simulink model "SimulationModel"  (R2017b)
settings: Solver=ode4  StartTime=0.0  StopTime=inf  RelTol=1e-3
PreLoadFcn:
  | addLibrariesInPath('sim')
PostLoadFcn:
  | loadRobotParameters
StartFcn:
  | simApp = SimDisplay.getInstance;
  | simApp.reset;
  | simApp.TrackView.setup(double(SitesPositions), ObstaclesPositions,ObstaclesVertices,ObstaclesEdges);
values from neighbouring files (symbols this model uses):
  AngularSpeed = 300    [loadRobotParameters.m]
  AxleLength = 16.7    [loadRobotParameters.m]
  DISTANCE_APPROACH = 45    [loadRobotParameters.m]
  DISTANCE_MAX = 200    [loadRobotParameters.m]
  DISTANCE_PARKING = 10    [loadRobotParameters.m]
  do_one_run = true    [loadRobotParameters.m]
  EncL_init = 0    [loadRobotParameters.m]
  EncR_init = 0    [loadRobotParameters.m]
  EncRes = 636    [loadRobotParameters.m]
  lcam = [21, 90]    [loadRobotParameters.m]
  motorL = [-967.207000 -900.359000 -783.375000 -618.344000 -325.884000 -0.000000 0.000000 325.884000 618.344000 783.375000 900.359000 967.207000 ]    [loadRobotParameters.m]
  motorR = [-937.961000 -850.223000 -768.752000 -618.344000 -302.905000 -0.000000 0.000000 302.905000 618.344000 768.752000 850.223000 937.961000 ]    [loadRobotParameters.m]
  motorX = [-100.000000 -90.000000 -70.000000 -50.000000 -30.000000 -27.000000 27.000000 30.000000 50.000000 70.000000 90.000000 100.000000 ]    [loadRobotParameters.m]
  pcam = [24, 100]    [loadRobotParameters.m]
  RADIUS_TARGET = 5    [loadRobotParameters.m]
  S_ROT = 10    [loadRobotParameters.m]
  SPEED_APPROACH = 15    [loadRobotParameters.m]
  SPEED_BACK = 5    [loadRobotParameters.m]
  SPEED_NORMAL = 30    [loadRobotParameters.m]
  startPos = single([150 150])    [loadRobotParameters.m]
  TauMotor = 0.1    [loadRobotParameters.m]
  TH1 = 5    [loadRobotParameters.m]
  TH2 = 15    [loadRobotParameters.m]
  theta0 = 0    [loadRobotParameters.m]
  Ts = 0.1    [loadRobotParameters.m]
  WAIT_TIME = 4    [loadRobotParameters.m]
  WheelRadius = 7/2    (= 3.5)    [loadRobotParameters.m]
undefined symbols (not defined in the file or in its folder): ObstaclesEdges, ObstaclesVertices, SitesPositions
libraries: simulink_extras x2, simulink x2, Fuzzy_Type2_Lib x1, realtime_pacer_lib x1, cstblocks x1
(part 2 of 2)

== stateflow chart SimulationModel/RobotModel/Controller/FeedbackController/ControllerModesDistance ==
  state CurrentMove [parallel]
    settings: executionOrder=1
    state Normal
      entry:
      EncodersZero = Encoders;
      entry,during:
      CurrentDistance = CurrentMoveFcn(Encoders,EncodersZero);
    state distance = CurrentMoveFcn(enc,zero) [function]
    (default) -> Normal
    Normal -> Normal : Reset
  state ModeControl [parallel]
    settings: executionOrder=2
    state SpeedControl
      entry:
      CurrentMove.Reset;
      ResetDistancePI;
      DistanceError = Cmd.Position;
      PrevDistance = CurrentDistance;
      during:
      DistanceError = (Cmd.Position - (CurrentDistance-PrevDistance)/Ts);
      PrevDistance = CurrentDistance;
    state DistanceControl
      entry:
      CurrentMove.Reset;
      ResetDistancePI;
      entry,during:
      DistanceError = Cmd.Position - CurrentDistance;
    (default) -> (junction 73)
    (junction 73) -> (junction 72) [order 1] : [Cmd.Mode == EMode.SPEED]
    (junction 73) -> DistanceControl [order 2]
    (junction 72) -> SpeedControl
    SpeedControl -> DistanceControl : [Cmd.Mode == EMode.DISTANCE]
    DistanceControl -> SpeedControl : [Cmd.Mode == EMode.SPEED]
  state ResetIntegrator [parallel]
    settings: executionOrder=4
    (default) -> (junction 189) : {
        | PrevCmd = Cmd.Position;
        | PrevMode = Cmd.Mode;
        | }
    ResetIntegrator -> (junction 189)
    (junction 189) -> (junction 192) [order 1] : [Cmd.Mode ~= PrevMode]
    (junction 189) -> (junction 179) [order 2]
    (junction 192) -> (junction 185)
    (junction 179) -> (junction 185) [order 1] : [sign(Cmd.Position) ~= sign(PrevCmd)]
    (junction 179) -> (junction 188) [order 2]
    (junction 185) -> (junction 187) : {
        | ResetDistancePI;
        | }
    (junction 187) -> (junction 188)
    (junction 188) -> (junction 181) : {
        | PrevCmd = Cmd.Position;
        | PrevMode = Cmd.Mode;
        | }
  state ErrorInitialCondition [parallel]
    settings: executionOrder=3
    (default) -> (junction 170)
    ErrorInitialCondition -> (junction 170)
    (junction 170) -> (junction 171) [order 1] : [abs(DistanceError) < 30 && ...
        | abs(Cmd.Angle) < 1 && ...
        | Cmd.Mode == EMode.SPEED]
    (junction 170) -> (junction 172) [order 2] : {
        | DistanceIC = single(0);
        | }
    (junction 171) -> (junction 173) : {
        | DistanceIC = 30 * sign(Cmd.Position) - DistanceError;
        | }
    (junction 173) -> (junction 172)
    (junction 172) -> (junction 174)
  data: enc function_input int32 size=2; zero function_input int32 size=2; distance function_output; EncodersZero local int32 size=2; PrevDistance local; PrevCmd local; PrevMode local; Encoders input int32 size=2; CurrentDistance local single; DistanceError output single size=1; Cmd input Bus: bus_Command; Ts parameter; DistanceIC output
  events: Reset local FUNCTION_CALL_EVENT; ResetDistancePI output EITHER_EDGE_EVENT

== stateflow chart SimulationModel/Scoring/Referee/Referee ==
  state Standby
    entry:
    numTargets = size(SitesPositions,1);
    targetsFound = false(size(SitesPositions,1),1);
    timeLastTargetFound = 0;
    elapsedTime = 0;
    numTargetsFound = 0;
    allowedRunTime = 180;
    startingRadius = 10;
    targetBoundaryRadius = 7;
    statTimeReq = 2.5;
  state Running
    entry: startTiming;
    during:
    elapsedTime = getTiming;
    [nearLocation, currentTarget] = testIfNearLocation(robotPosition, SitesPositions, targetBoundaryRadius);
    state NearLocation
      entry: snapshotTime = elapsedTime;
    state Roaming
    Roaming -> NearLocation : [nearLocation == true]
    (default) -> Roaming
    NearLocation -> Roaming [order 2] : [nearLocation == false]
    NearLocation -> (junction 43) [order 1] : [(elapsedTime - snapshotTime) > statTimeReq]
    (junction 44) -> Roaming
    (junction 43) -> (junction 44) : {[targetsFound, timeLastTargetFound] = ...
        | updateTargetsFound(targetsFound, currentTarget, timeLastTargetFound,elapsedTime);
        | numTargetsFound = sum(targetsFound);}
  state Finished
  (default) -> Standby
  Finished -> Standby : [StartFlag == false]
  Standby -> Running : [StartFlag == true &&...
      | distancefrom(robotPosition, startPos) < startingRadius ]
  Running -> Standby [order 2] : [StartFlag == false]
  Running -> Finished [order 1] : [numTargetsFound == numTargets ||...
      |  elapsedTime >= allowedRunTime-sqrt(eps)]
  data: et function_output; tfound_in function_input; currentT function_input; tfound_out function_output; lastTime_in function_input; lastTime_out function_output; time function_input; robotPos function_input; targetPos function_input; proximityVal function_input; nearLoc function_output; currentLoc function_output; pos function_input; x0 function_input; d function_output; startPos parameter; allowedRunTime local; statTimeReq local; startingRadius local; robotPosition input; targetBoundaryRadius local; StartFlag input; SitesPositions parameter; timeLastTargetFound output; nearLocation local; numTargetsFound local; elapsedTime output; numTargets local; currentTarget local; targetsFound output; snapshotTime local; local_t local =0; sim_time input
  function startTiming:
    | function startTiming
    | global local_t sim_time
    | 
    | if strcmp(coder.target,'rtw')
    |     coder.ceval('tic',int32(2));
    | else
    |     local_t = sim_time;
    | end
  function et = getTiming:
    | function et = getTiming
    | global sim_time local_t
    | 
    | lt = 0;
    | 
    | if strcmp(coder.target,'rtw')
    |     coder.ceval('toc',coder.wref(lt),int32(2));
    | else
    |     lt = sim_time - local_t;
    | end
    | 
    | et = lt;
  function [tfound_out, lastTime_out] = updateTargetsFound(tfound_in, currentT, lastTime_in, time):
    | function [tfound_out, lastTime_out] = updateTargetsFound(tfound_in, currentT, lastTime_in, time)
    | 
    | if any(tfound_in & currentT) %is this an existing target
    |     lastTime_out = lastTime_in;
    | else
    |     lastTime_out = time;
    | end
    | 
    | tfound_out = tfound_in | currentT; %update list of found targets
  function [nearLoc, currentLoc] = testIfNearLocation(robotPos, targetPos, proximityVal):
    | function [nearLoc, currentLoc] = testIfNearLocation(robotPos, targetPos, proximityVal)
    | %#codegen
    | delta = bsxfun(@minus, targetPos, robotPos);
    | dist = sum(delta.^2,2);
    | 
    | currentLoc = dist <= proximityVal^2;
    | nearLoc = any(currentLoc);
  function d = distancefrom(pos,x0):
    | function d = distancefrom(pos,x0)
    | d = sqrt(sum((pos-x0).^2));

== matlab function SimulationModel/Scoring/FigureOutput/call_plotFigure ==
  data: X input; SitesPositions parameter; T_found input; t_last input; t input; T_located input; pcam parameter; lcam parameter; robotheta input; ArmAngleEstimated input; ArmAngleCommand input; DisplayPositions input
function fcn(X, SitesPositions, T_found, t_last, t, T_located,pcam,lcam,robotheta,...
    ArmAngleEstimated, ArmAngleCommand, DisplayPositions)
coder.extrinsic('plotFigure');

plotFigure(X, SitesPositions, T_found, t_last, t, T_located,pcam,lcam,robotheta,...
    single(ArmAngleEstimated), single(ArmAngleCommand), DisplayPositions);

== matlab function SimulationModel/RobotModel/Robot/Sensors Camera_Distance/Camera/relative_to_targets ==
  data: robotPos input size=[1 2]; robotTheta input size=1; dist output; bear output; SitesPositions parameter single; ObstaclesVertices parameter; ObstaclesEdges parameter; pcam parameter; lcam parameter
 function [dist,bear] = targets(robotPos,robotTheta,SitesPositions,ObstaclesVertices, ObstaclesEdges, pcam,lcam)
%#codegen
%% TARGETS Returns distance and bearing for each target relative tos robot
%
% Distances and positions are in cm
% Angles are in degrees
%
% Inputs
%   - hCam: Cam height (from ground)
%   - targetsPos: Position of targets (X,Y)
%   - robotPos: Robot position (X,Y)
%   - robotTheta: Robot angle
%
% Outputs
%   - dist (array nx1 with n=nb targets): Distances for each target,
%       if a target cannot be seen by the camera associated distance
%       is equal to -1
%   - bearing (array nx1 with n=nb targets): Angles for each target,
%       if a target cannot be seen by the camera associated angle is
%       equal to -1
%

% Get camera field of vision
% [pcam,lcam]=camera(hCam);
% betaCam = 21 ;
% etaCam = 27 ;
% [pcam, lcam] = cameraAnalytic(hCam,90-alphaCam, betaCam, etaCam);

% Convert target position to robot reference
[x,y] = world2robot(robotPos(1),robotPos(2),robotTheta,SitesPositions(:,1),SitesPositions(:,2));

% Convert Obstacles positions to robot reference
[vx,vy] = world2robot(robotPos(1),robotPos(2),robotTheta,ObstaclesVertices(:,1),ObstaclesVertices(:,2));

% Get left and right detector indicators
%[leftFlag, rightFlag] = isThereSomething(vx, vy, obstaclesEdges);

% Get distance and bearing for each point relative to robot
[distance,bearing] = isincamera(pcam,lcam,x,y,vx,vy,ObstaclesEdges);

% sort by descending order and return 6 elements
[distance,idxsort] = sort(distance,'descend');
bearing = bearing(idxsort);
if length(distance)<6
    dist = [distance;zeros(6-length(distance),1)];
    bear = [bearing;zeros(6-length(bearing),1)] ;
else
    dist = distance(1:6);
    bear = bearing(1:6);
end

end

function [x_new,y_new]=world2robot(x_robot,y_robot,theta_robot,x_world,y_world)
% WORLD2ROBOT Convert coordinates from world to robot
%
% Inputs
%   - x_robot: Robot X position (in world reference)
%   - y_robot: Robot Y position (in world reference)
%   - theta_robot: Robot angle  (in world reference)
%   - x_world: X value(s) to convert (in world reference)
%   - y_world: Y value(s) to convert (in world reference)
%
% Outpus
%   - x_new: Point(s) coordinate (X) in robot reference
%   - y_new: Point(s) coordinate (Y) in robot reference

% Translate coordinates reference
x_dif=x_world-x_robot;
y_dif=y_world-y_robot;

% Rotate coordinates reference
% x_new=x_dif*cosd(theta_robot)-y_dif*sind(theta_robot);
% y_new=x_dif*sind(theta_robot)+y_dif*cosd(theta_robot);
x_new = cosd(theta_robot)*x_dif + sind(theta_robot)*y_dif;
y_new = cosd(theta_robot)*y_dif - sind(theta_robot)*x_dif;
% see http://www.mathematics-online.org/inhalt/aussage/aussage444/

% TODO We have identified that the sign of converted coordinates is the
% opposite of the expected but we don't have an explanation for that
% x_new = -x_new;
% y_new = -y_new;

end

function [dist,bearing]=isincamera(p,l,x,y,vx,vy,OE)
%% ISINCAMERA Distance and angle from current robot position
%
% Inputs
%   - p (2 elements vector): Minimal and maximal depth for camera (Y axis)
%   - l (2 elements vector): Minimal and maximal width for camera (X axis)
%   - x (vector): X coordinate of point(s)
%   - y (vector): Y coordinate of point(s)
%
% Outputs
%   - dist (vector): Distance of each point from camera (robot), -1 if
%       point cannot be seen by camera.
%   - bearing (vector): Angle of each point from camera (robot), -1 if
%       point cannot be seen by camera.
%

% Calculate coefficients for lines that defines the camera field of vision
% Field vision limits in Y axis are constants (y = p(1) or y = p(2))
% c1=polyfit(p(1:2),[-l(1)/2 -l(2)/2],1);
% c2=polyfit(p(1:2),[l(1)/2 l(2)/2],1);

% To be visible a point must match all the following criterion
%   - Y >= minimal depth
%   - Y <= maximal depth
%   - X >= - (width for current Y) / 2
%   - X <=   (width for current Y) / 2
%

%isvisible = y>=p(1) & y<=p(2) & (x>=polyval(c1,y) & x<=polyval(c2,y));
% isvisible = x>=p(1) & x<=p(2) & (y>=polyval(c1,x) & y<=polyval(c2,x));

%TTx = [p(1) p(2) p(2) p(1)]' ;
%TTy = [l(1)/2 l(2)/2 -l(2)/2 -l(1)/2]' ;
%TTx = [[p(1); p(2); p(1)] [p(1); p(2); p(2)]];
%TTy = [[l(1)/2; l(2)/2; -l(1)/2] [-l(1)/2; l(2)/2; -l(2)/2]];
TTx = [p(1); p(2); p(2); p(1)];
TTy = [l(1)/2; l(2)/2; -l(2)/2; -l(1)/2];

[vpX, vpY] = CastRays(0, 0, [vx vy], OE);
vpX = vpX(2:end,:);
vpX = vpX(:);
vpY = vpY(2:end,:);
vpY = vpY(:);

%dis = simDisplay.getInstance;
%patch(vpX, vpY, zeros(size(vpX)), 'Parent', dis.TrackView.Axes);


isvisible = true(size(x));
for k=1:length(isvisible)
    isvisible(k) = any(myInpolygon(x(k), y(k), TTx, TTy)) && ...
        any(myInpolygon(x(k), y(k), vpX, vpY));
%     isvisible(k) = any(inTriangle(x(k), y(k), TTx, TTy)) &&...
%         any(inTriangle(x(k), y(k), vpX, vpY));
end

% Calculate distance and bearing for all points
dist = sqrt(x.^2 + y.^2);
% bearing = atan2d(y,x);
bearing = atan2d(x,-y)-90;

% Replace values by -1 for points that are not visible
dist(~isvisible) = 0;
bearing(~isvisible) = 0;

end

function [vpX, vpY] = CastRays(x, y, vertices, edges)
% Cast rays

vertices = [vertices zeros(length(vertices),5)];
% Compute relative cartesian coordinates
vertices(:,3) = vertices(:,1) -...
    x;

vertices(:,4) = vertices(:,2) -...
    y;


% Compute relative polar coordinates
[vertices(:,5), vertices(:,6)] =...
    cart2pol(vertices(:,3), vertices(:,4));

vertices(:,5) = mod(vertices(:,5), 2*pi);


% Sort rows by angle and get reverse permutation
[vertices, ind] = sortrows(vertices, 5);

[~, ind] = sort(ind, 'ascend');


% Modify the edges indices accordingly
edges(:,1) = ind(edges(:,1));

edges(:,2) = ind(edges(:,2));


% Ensure that the left vertex of each edge is on the left
Tdiff = vertices(edges(:,1),5) -...
    vertices(edges(:,2),5);

ind = xor(Tdiff < 0, abs(Tdiff)>pi);

edges(ind, [1 2]) =...
    edges(ind, [2 1]);

vpX = zeros(3, size(vertices,1));
vpY = zeros(3, size(vertices,1));


% Loop over each vertex and get the left vertex of the
% right triangle and the right edge of the left triangle
for ray = 1:size(vertices,1)
    
    % Find edges that cross the ray
    TdiffL = vertices(edges(:,1),5) -...
        vertices(ray,5);
    TdiffR = vertices(ray,5) -...
        vertices(edges(:,2),5);
    intersects = find(xor(TdiffL >= 0, abs(TdiffL)>pi) &...
        xor(TdiffR >= 0, abs(TdiffR)>pi));
    
    
    % Compute intersection coordinates
    [~, ~, interX, interY] = lineSegmentsIntersection(x, y, vertices(ray,1),...
        vertices(ray,2), vertices(edges(intersects,1),1),...
        vertices(edges(intersects,1),2), vertices(edges(intersects,2),1),...
        vertices(edges(intersects,2),2));
    
    
    % Sort the intersections (coordinates and index of the
    % edges) by distance to viewpoint
    [~, dist2vp] = cart2pol(interX - x, interY - y);
    
    [~,ind] = sort(dist2vp, 'ascend');
    
    intersects = intersects(ind);
    
    
    % Pick the first intersection, with the exception that it
    % must not be a right edge for the left triangle or a left
    % edge for the right triangle. Assign the result
    leftInd = find(edges(intersects,2) ~= ray, 1, 'first');
    rightInd = find(edges(intersects,1) ~= ray, 1, 'first');
    if isempty(leftInd)
        leftInd = 1;
    end
    if isempty(rightInd)
        rightInd = 1;
    end
    rightInd = rightInd(1);
    leftInd = leftInd(1);
    
    vpX(1,ray) = x;
    vpY(1,ray) = y;
    
    vpX(2,ray) = interX(ind(rightInd));
    vpY(2,ray) = interY(ind(rightInd));
    
    indBack = mod(ray-2, size(vertices,1))+1;
    vpX(3,indBack) = interX(ind(leftInd));
    vpY(3,indBack) = interY(ind(leftInd));
    
end

end

== matlab function SimulationModel/RobotModel/Robot/Sensors Camera_Distance/Camera/dist_bearing2locatedTargets ==
  data: robotPos input; dist input; locatedTargets output; bearing input; robotTheta input
function locatedTargets = fcn(robotPos, dist, bearing, robotTheta)
%#codegen

loc = dist > 0;

locatedTargetsX = zeros(size(dist));
locatedTargetsY = locatedTargetsX;

targetTheta = robotTheta + bearing(loc);

locatedTargetsX(loc) = robotPos(1) + dist(loc) .* cosd(targetTheta);
locatedTargetsY(loc) = robotPos(2) + dist(loc) .* sind(targetTheta);

locatedTargets = [locatedTargetsX, locatedTargetsY];

== stateflow chart SimulationModel/InputProcessing/Strategy ==
  settings: sampleTime=Ts
  state Process [parallel]
    settings: executionOrder=2
    state Init
      entry:
      [DistanceCameraTargetsFiltred , BearingCameraTargetsFiltred] =filter(DistanceCameraTargets ,BearingCameraTargets , RobotXY , RobotTheta , visitedX , visitedY);
    (default) -> Process.Init
    Process.Init -> Process.Init : after(0.2,sec)
  state Navigation [parallel]
    settings: executionOrder=1
    state Normal
      entry,during:
      Mode = EMode.SPEED;
      TranslationCmd = single(SPEED_NORMAL*isTranslation) ;
      RotationCmd = - single(0+rotationCorrection); % TODO : changer signe -
      % TODO : Optimer les types de données
    state GoToTarget
      state TargetInView
        %TODO : Optimisation et factorisation à faire
        entry:
        Mode = EMode.SPEED; % Commande en vitesse si loin
        RemainingDistance=single(DISTANCE_MAX);
        RemainingBearing=single(DISTANCE_MAX);
        RotationCmd=single(0); % freinage d'abord
        TranslationCmd=single(0);
        ResetEncoder;
        during:
        if  ~isempty(DistanceCameraTargetsFiltred(DistanceCameraTargetsFiltred>0)) %TODO ;  A supprimer pour éviter les oscilliations ?
        indClosestTarget = ((find(DistanceCameraTargetsFiltred ==  min(DistanceCameraTargetsFiltred(DistanceCameraTargetsFiltred>0) ) ) ));
        ind = min (indClosestTarget);
        DistanceToTarget=single(DistanceCameraTargetsFiltred(ind));
        TranslationCmd= single(SPEED_APPROACH); % Fichier de conf
        RemainingDistance=DistanceToTarget;
        BearingToTarget= -single(BearingCameraTargetsFiltred(ind));
        RotationCmd=BearingToTarget;
        RemainingBearing= BearingToTarget;
        end
      state TargetHidden
        entry:
        Mode = EMode.DISTANCE; % Commande en position
        TranslationCmd=RemainingDistance ; % Pour etre sous le cadre
        RotationCmd=RemainingBearing;
        ResetEncoder;
        during:
        RemainingDistance = DistanceToTarget - CurrentDistance;
      (default) -> TargetInView
      TargetInView -> TargetHidden [order 2] : [ RemainingDistance < (DISTANCE_APPROACH) ]
    state Init
      entry,during:
      spotVisited=double(0);
      visitedX= zeros(1, 20);
      visitedY= zeros(1, 20);
      TranslationCmd=single(0);
    state GoBack [commented out]
      entry,during:
      TranslationCmd=single(-SPEED_BACK);
      RotationCmd=single(0);
    state SearchTargetAround
      state WaitRight
        entry:
        TranslationCmd=single(0);
        RotationCmd=single(0);
      state GoBackToZero
        entry:
        TranslationCmd=single(0);
        RotationCmd= single(S_ROT);
        ResetEncoder;
      state SearchFirstRightTarget
        entry:
        TranslationCmd=single(0);
        RotationCmd=single(-S_ROT);
        ResetEncoder;
      state SearchLeftTarget
        entry:
        Mode = EMode.SPEED;
        initTheta=double(RobotTheta);
        TranslationCmd=single(0);
        RotationCmd=single(S_ROT );
        ResetEncoder;
      state WaitLeft
        entry:
        TranslationCmd=single(0);
        RotationCmd=single(0);
      SearchFirstRightTarget -> WaitRight : [CurrentBearing>180 || ...
          |  abs(rotationCorrection) > TH1 ]
      WaitRight -> GoBackToZero : [after(1,sec) || ...
          |   abs(rotationCorrection) > TH1 ]
      WaitLeft -> SearchFirstRightTarget : [after(1,sec) || ...
          |  abs(rotationCorrection) > TH1 ]
      (default) -> SearchLeftTarget
      SearchLeftTarget -> WaitLeft : [CurrentBearing<-90 || ...
          |  abs(rotationCorrection) > TH1]
    state Wait_for_scoring
      entry:
      Mode = EMode.SPEED;
      out = single(0);
      if min(sqrt( (visitedX-RobotXY(1)).^2 + (visitedY-RobotXY(2)).^2)) > (RADIUS_TARGET)
      spotVisited = spotVisited + 1;
      visitedX(spotVisited) = RobotXY(1);
      visitedY(spotVisited) = RobotXY(2);
      TranslationCmd = single(0);
      RotationCmd = single(0);
      else
      out=single(1);
      end;
      ResetEncoder;
    TargetInView -> Normal [order 1] : [max(DistanceCameraTargetsFiltred) == 0]
    GoBackToZero -> Normal : [abs(mod(RobotTheta -  initTheta, 2*pi)) < ...
        | 0.2]
    Normal -> GoToTarget : [max(DistanceCameraTargetsFiltred) ~= 0]
    (default) -> Navigation.Init
    Navigation.Init -> GoToTarget [order 1] : [max(DistanceCameraTargetsFiltred) ~= 0]
    Navigation.Init -> SearchTargetAround [order 2] : after(1, sec)
    GoBack -> GoBackToZero [commented out] : [abs(rotationCorrection) < TH2 ]
    SearchTargetAround -> GoBack [commented out] : [abs(rotationCorrection) > (TH2-1) ]
    SearchTargetAround -> GoToTarget : [max(DistanceCameraTargetsFiltred) ~= 0]
    GoToTarget -> Wait_for_scoring : [ RemainingDistance < (DISTANCE_PARKING) ]
    Wait_for_scoring -> SearchTargetAround : [after(WAIT_TIME,sec) || out == 1]
  data: DistanceCamera function_input; DistanceCameraFiltred function_output; BearingCamera function_input; RobXY function_input; RobotTh function_input; VisX function_input; VisY function_input; BearingCameraFiltred function_output; RotationCmd output single size=1; TranslationCmd output single size=1; DistanceCameraTargets input int16; BearingCameraTargets input int8; CurrentDistance input single; CurrentBearing input single; BearingToTarget local single; DistanceToTarget local single; ind local; rotationCorrection input; RobotXY input size=[1 2]; targetX local size=[1 6]; targetY local size=[1 6]; spotVisited local; i local =0; Yt local single; ThetaT local single; Xt local single; visitedX local size=[1 20]; visitedY local size=[1 20]; D local single size=[1 20]; BearingCameraTargetsFiltred local; DistanceCameraTargetsFiltred local; RobotTheta input single size=1; out local single; initTheta local; isTranslation input; indClosestTarget local size=[1,6]; Mode output Enum: EMode; RemainingBearing local single; RemainingDistance local single; SPEED_NORMAL parameter; S_ROT parameter; SPEED_BACK parameter; TH1 parameter; WAIT_TIME parameter; SPEED_APPROACH parameter; TH2 parameter; DISTANCE_MAX parameter; DISTANCE_APPROACH parameter; DISTANCE_PARKING parameter; RADIUS_TARGET parameter
  events: ResetEncoder output EITHER_EDGE_EVENT
  function [DistanceCameraFiltred , BearingCameraFiltred] =filter(DistanceCamera ,BearingCamera , RobXY , RobotTh , VisX , VisY):
    | function [DistanceCameraFiltred , BearingCameraFiltred] =filter(DistanceCamera ,BearingCamera , RobXY , RobotTh , VisX , VisY)
    |  
    | DistanceCameraFiltred = double(DistanceCamera);
    | BearingCameraFiltred = double(BearingCamera);
    | for i =1:length(DistanceCameraFiltred)
    |     if DistanceCameraFiltred(i) ~= 0
    |         ThetaT=single(BearingCamera(i))*single(pi/180) + RobotTh;
    |         Xt=RobXY(1) + single(DistanceCamera(i))*cos(ThetaT);
    |         Yt=RobXY(2) + single(DistanceCamera(i))*sin(ThetaT);
    |         D=sqrt( (VisX-Xt).^2 + (VisY-Yt).^2);
    |         if min(D) < 40
    |             DistanceCameraFiltred(i) = 0;
    |             BearingCameraFiltred(i) = 0;
    |         end
    |     end
    | end
    | end

== matlab function SimulationModel/RobotModel/Robot/Sensors Camera_Distance/Distance_sensor/arm_distance ==
  data: robotPos input size=[1 2]; robotTheta input size=1; armAngle input; ObstaclesVertices parameter; ObstaclesEdges parameter; armDist output
 function armDist  = targets(robotPos,robotTheta,armAngle,ObstaclesVertices, ObstaclesEdges)
%#codegen
%% TARGETS Returns distance and bearing for each target relative tos robot
%
% Distances and positions are in cm
% Angles are in degrees
%
% Inputs
%   - hCam: Cam height (from ground)
%   - targetsPos: Position of targets (X,Y)
%   - robotPos: Robot position (X,Y)
%   - robotTheta: Robot angle
%
% Outputs
%   - dist (array nx1 with n=nb targets): Distances for each target,
%       if a target cannot be seen by the camera associated distance
%       is equal to -1
%   - bearing (array nx1 with n=nb targets): Angles for each target,
%       if a target cannot be seen by the camera associated angle is
%       equal to -1
%

% Get camera field of vision
% [pcam,lcam]=camera(hCam);
% betaCam = 21 ;
% etaCam = 27 ;
% [pcam, lcam] = cameraAnalytic(hCam,90-alphaCam, betaCam, etaCam);

% Convert Obstacles positions to robot reference
[vx,vy] = world2robot(robotPos(1),robotPos(2),robotTheta,ObstaclesVertices(:,1),ObstaclesVertices(:,2));

[~, ~, ~, ~, ua, ub] = lineSegmentsIntersection(0, 0,...
    cosd(single(armAngle)), sind(single(armAngle)), vx(ObstaclesEdges(:,1)),...
    vy(ObstaclesEdges(:,1)), vx(ObstaclesEdges(:,2)), vy(ObstaclesEdges(:,2)));

isOnRange = (ua >= 10) & (ua <= 80) & (ub >= 0) & (ub <= 1);

if nnz(isOnRange)==0
    armDist = int8(-1);
else
    armDist = int8(min(ua(isOnRange)));
end


end

function [x_new,y_new]=world2robot(x_robot,y_robot,theta_robot,x_world,y_world)
% WORLD2ROBOT Convert coordinates from world to robot
%
% Inputs
%   - x_robot: Robot X position (in world reference)
%   - y_robot: Robot Y position (in world reference)
%   - theta_robot: Robot angle  (in world reference)
%   - x_world: X value(s) to convert (in world reference)
%   - y_world: Y value(s) to convert (in world reference)
%
% Outpus
%   - x_new: Point(s) coordinate (X) in robot reference
%   - y_new: Point(s) coordinate (Y) in robot reference

% Translate coordinates reference
x_dif=x_world-x_robot;
y_dif=y_world-y_robot;

% Rotate coordinates reference
% x_new=x_dif*cosd(theta_robot)-y_dif*sind(theta_robot);
% y_new=x_dif*sind(theta_robot)+y_dif*cosd(theta_robot);
x_new = cosd(theta_robot)*x_dif + sind(theta_robot)*y_dif;
y_new = cosd(theta_robot)*y_dif - sind(theta_robot)*x_dif;
% see http://www.mathematics-online.org/inhalt/aussage/aussage444/

% TODO We have identified that the sign of converted coordinates is the
% opposite of the expected but we don't have an explanation for that
% x_new = -x_new;
% y_new = -y_new;

end
